simulink model "MPC_point7"  (R2024b)
settings: Solver=FixedStepDiscrete  StartTime=0.0  StopTime=100  FixedStep=Ts  RelTol=1e-3  EnableMultiTasking=on
values from neighbouring files (symbols this model uses):
  A_tilde = [Az, zeros(num,1) ... (first row only)    [main.m]
  B_tilde = [Bz; -Cz*Bz]    [main.m]
  C_state = eye(12)    [main.m]
  D_state = zeros(12, 1)    [main.m]
  QMPC = Q_tilde    [main.m]
  R_LQ = r    (= 1e-05)    [main.m]
  S_tilde = zeros(13)    [main.m]
  Ts = 0.1    [main.m]    (also in point7.m)
  umax = +15    (= 15)    [main.m]
  umin = -15    [main.m]
  x0 = [3,0,3,0,3,0,3,0,3,0,3,0]    [main.m]
  Ybar = 1    [main.m]
undefined symbols (not defined in the file or in its folder): Az_bis, Bz_bis, Cz, DiscIntNeverNeededParam, mympc_velocityform
libraries: simulink x1
settings Model: Creator=Mirko  LastModifiedBy=faiol
settings SolverCC: AlgebraicLoopSolver=TrustRegion
settings DataIOCC: LimitDataPoints=on  SaveFormat=Array  SignalLoggingSaveFormat=ModelDataLogs  ReturnWorkspaceOutputs=off
settings OptimizationCC: ExpressionDepthLimit=2147483647  LifeSpan=inf
settings DebuggingCC: UnderspecifiedInitializationDetection=Classic  MergeDetectMultiDrivingBlocksExec=none  SolverPrmCheckMsg=warning  FcnCallInpInsideContextMsg=warning  UnconnectedInputMsg=warning  UnconnectedOutputMsg=warning  UnconnectedLineMsg=warning  StateNameClashWarn=warning  SFUnexpectedBacktrackingDiag=warning  SFNoUnconditionalDefaultTransitionDiag=warning  SFExecutionAtInitializationDiag=none  ArithmeticOperatorsInVariantConditions=warning
settings HardwareCC: ProdBitPerPointer=32  ProdBitPerSizeT=32  ProdBitPerPtrDiffT=32  ProdLargestAtomicFloat=None  ProdIntDivRoundTo=Undefined  ProdEndianess=Unspecified  ProdWordSize=32  ProdHWDeviceType=32-bit Generic
settings ModelReferenceCC: EnableRefExpFcnMdlSchedulingChecks=on  PropagateSignalLabelsOutOfModel=off
settings SFSimCC: SimUseLocalCustomCode=off  CustomCodeUndefinedFunction=UseInterfaceOnly
settings RTWCC: RTWUseLocalCustomCode=off  GPUComputeCapability=3.5  DLArmComputeVersion=19.05
settings CodeAppCC: StateflowObjectComments=on
settings GRTTargetCC: TargetLangStandard=C89/C90 (ANSI)
settings ConfigComp: CovMetricSettings=dw  CovSaveCumulativeToWorkspaceVar=on  CovSaveSingleToWorkspaceVar=on  CovExternalEMLEnable=off  CovSFcnEnable=off

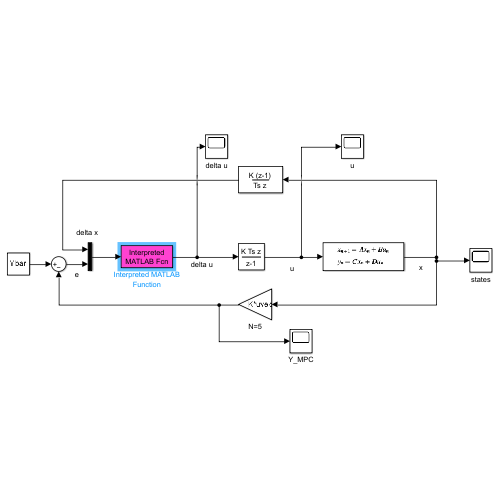
[thumbnail: Simulink's stored preview of the top-level diagram]
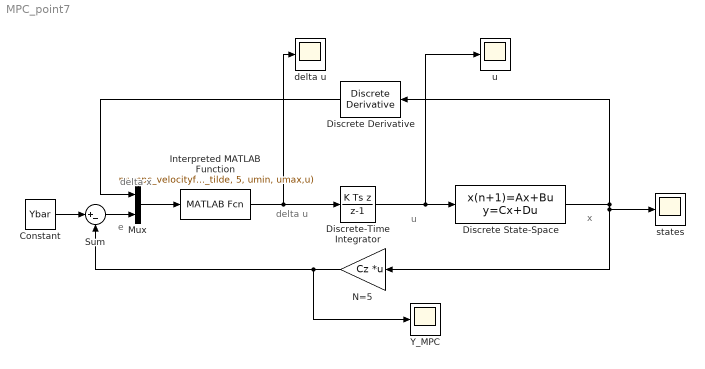
== system MPC_point7 ==
  note: x
  note: u
  note: delta u
  note: e
  note: delta x
  Constant : Constant  Value=Ybar
  Discrete Derivative : simulink/Discrete/Discrete Derivative  gainval=1.0  ICPrevScaledInput=0.0  OutMin=[]  OutMax=[]  OutDataType=fixdt(1, 16)  OutScaling=2^-10  DoSatur=off
  Discrete State-Space : DiscreteStateSpace  A=Az_bis  B=Bz_bis  C=C_state  D=D_state  InitialCondition=x0  SampleTime=Ts
  Discrete-Time Integrator : DiscreteIntegrator  IntegratorMethod=Integration: Backward Euler  SampleTime=Ts  ICPrevOutput=DiscIntNeverNeededParam  ICPrevScaledInput=DiscIntNeverNeededParam
  Interpreted MATLAB Function : MATLABFcn  MATLABFcn=mympc_velocityform(A_tilde, B_tilde, QMPC, R_LQ, S_tilde, 5, umin, umax,u)  OutputDimensions=1
  Mux : Mux  Inputs=2
  N=5 : Gain  Gain=Cz  Multiplication=Matrix(K*u) (u vector)
  Sum : Sum  Inputs=|+-
  Y_MPC : Scope
  delta u : Scope
  states : Scope
  u : Scope
  wires:
  N=5/1 -> Y_MPC/1, Sum/2
  Mux/1 -> Interpreted MATLAB Function/1
  Discrete Derivative/1 -> Mux/1
  Sum/1 -> Mux/2
  Interpreted MATLAB Function/1 -> delta u/1, Discrete-Time Integrator/1
  Discrete-Time Integrator/1 -> u/1, Discrete State-Space/1
  Discrete State-Space/1 -> N=5/1, states/1, Discrete Derivative/1
  Constant/1 -> Sum/1
